simulink model "BatteryModel"  (R2025a)
settings: Solver=ode4  StartTime=startTime  StopTime=stopTime  FixedStep=600  RelTol=1e-3  EnableMultiTasking=on
PreLoadFcn:
  | load('parameters.mat'); load('temperature.mat'); load('powerDemand.mat'); ES.SoE_init = 0.5; startTime = 0; stopTime = 86400; ES.seriesCells = 84; ES.parallCells = 5;
StopFcn:
  | figure('Name', 'Battery Performance Dashboard', 'NumberTitle', 'off'); load('powerDemand.mat', 'powerDemand'); subplot(1,3,1); stairs([0:10:1430]/60, powerDemand/1e3, 'k-', 'linewidth', 2, 'DisplayName', 'Demand Track'); hold on; try stairs(tout/3600, actualPowerDrawn/1e3, 'r-', 'LineWidth', 1); catch; end; xlabel('Time [h]'); ylabel('Power [kW]'); grid on; title('Power Flux'); subplot(1,3,2); try stairs(tout/3600, esSOC*100, 'color', [0.9290 0.6940 0.1250], 'linewidth', 2); catch; end; xlabel('Time [h]'); ylim([0 110]); ylabel('% SOC'); grid on; title('Pack Energy Level'); subplot(1,3,3); try stairs(tout/3600, cellCapacity./cellCapacity(1)*100, 'k-', 'linewidth', 2); catch; end; xlabel('Time [h]'); ylabel('% SOH'); grid on; title('State of Health');
values from neighbouring files (symbols this model uses):
  ECM =     [matlab.mat]    (also in parameters.mat)
  ES =     [matlab.mat]    (also in parameters.mat)
  powerDemand = [230 3117.09108838 230 3802.27406847 230 230 230 3183.29523095 230 230 3203.47775068 230 ... (144 elements, 144x1)]    [powerDemand.mat]
  tempCelcius = [22 21.579121106 21.1646131714 20.7563616064 22.9631354938 24.9321480764 24.4525353275 23.9803499415 23.5154583277 23.0577292983 22.6070340251 22.163245997 ... (144 elements, 144x1)]    [temperature.mat]
undefined symbols (not defined in the file or in its folder): DiscIntNeverNeededParam
libraries: simulink x2
settings Model: Creator=Mario  LastModifiedBy=franc
settings SolverCC: AlgebraicLoopSolver=TrustRegion
settings DataIOCC: LimitDataPoints=on  SaveFormat=Array  SignalLoggingSaveFormat=ModelDataLogs  ReturnWorkspaceOutputs=off
settings OptimizationCC: LifeSpan=inf
settings DebuggingCC: SignalInfNanChecking=error  ReadBeforeWriteMsg=DisableAll  WriteAfterWriteMsg=DisableAll  WriteAfterReadMsg=DisableAll  InheritedTsInSrcMsg=none  MultiTaskDSMMsg=none  MultiTaskCondExecSysMsg=none  ParameterPrecisionLossMsg=none  UnconnectedInputMsg=warning  UnconnectedOutputMsg=warning  UnconnectedLineMsg=warning  AllowSymbolicDim=off  SFUnexpectedBacktrackingDiag=warning  SFNoUnconditionalDefaultTransitionDiag=warning  SFExecutionAtInitializationDiag=none  ArithmeticOperatorsInVariantConditions=warning
settings HardwareCC: ProdBitPerPointer=32.0  ProdBitPerSizeT=32.0  ProdBitPerPtrDiffT=32.0  ProdLargestAtomicFloat=None  ProdIntDivRoundTo=Undefined  ProdEndianess=Unspecified  ProdWordSize=32.0  ProdHWDeviceType=32-bit Generic
settings ModelReferenceCC: UpdateModelReferenceTargets=IfOutOfDate  EnableRefExpFcnMdlSchedulingChecks=on  PropagateSignalLabelsOutOfModel=off
settings SFSimCC: SFSimEcho=off  SimUseLocalCustomCode=off  CustomCodeUndefinedFunction=UseInterfaceOnly
settings RTWCC: RTWUseLocalCustomCode=off  GPUComputeCapability=3.5  DLArmComputeVersion=19.05
settings CodeAppCC: StateflowObjectComments=on
settings GRTTargetCC: TargetLangStandard=C89/C90 (ANSI)
settings ConfigComp: CovMetricSettings=dw  CovSaveCumulativeToWorkspaceVar=on  CovSaveSingleToWorkspaceVar=on  CovExternalEMLEnable=off  CovSFcnEnable=off

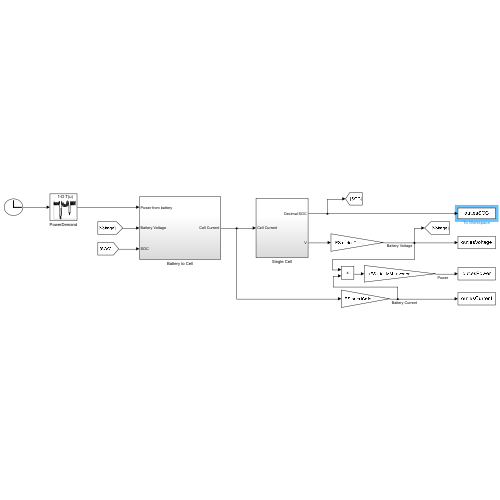
[thumbnail: Simulink's stored preview of the top-level diagram]
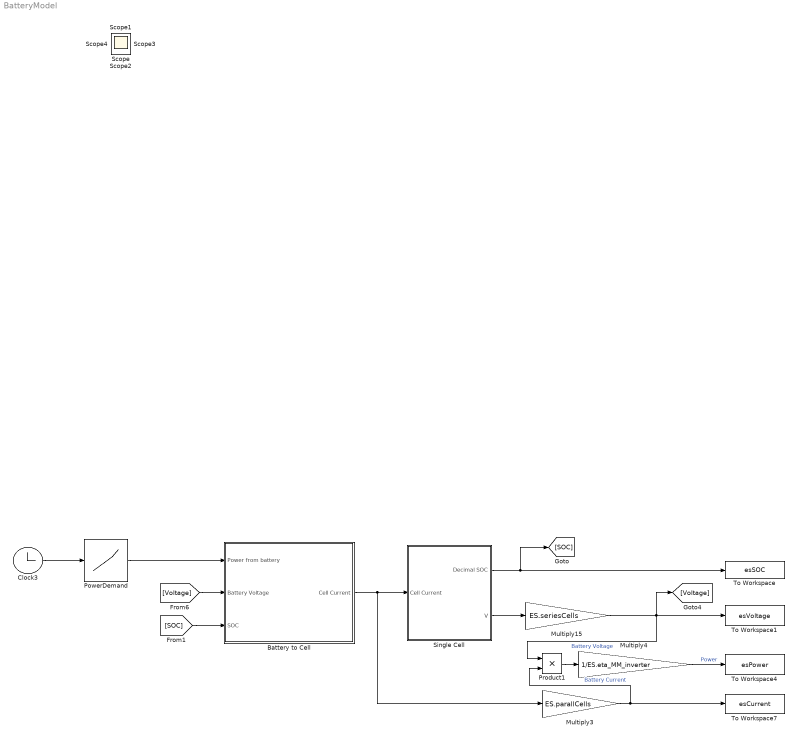
== system BatteryModel ==
  Battery to Cell : Subsystem
  Clock3 : Clock
  Multiply15 : Gain  Gain=ES.seriesCells
  Multiply3 : Gain  Gain=ES.parallCells
  Multiply4 : Gain  Gain=1/ES.eta_MM_inverter
  PowerDemand : Lookup_n-D  NumberOfTableDimensions=1  BreakpointsForDimension1=[0:600:85800]  Table=powerDemand  InternalRulePriority=Speed  RndMeth=Simplest
  Product1 : Product
  "Single Cell " : Subsystem
  To Workspace : ToWorkspace  VariableName=esSOC  SampleTime=-1
  To Workspace1 : ToWorkspace  VariableName=esVoltage  SampleTime=-1
  To Workspace4 : ToWorkspace  VariableName=esPower  SampleTime=-1
  To Workspace7 : ToWorkspace  VariableName=esCurrent  SampleTime=-1
  Scope{,1..4} (5 alike) : Scope
      Scope settings: ActiveDisplayYMinimum=-1  ActiveDisplayYMaximum=1
      Scope1 settings: ActiveDisplayYMinimum=-0.125  ActiveDisplayYMaximum=1.125  DataLoggingVariableName=ScopeData2
      Scope2 settings: ActiveDisplayYMinimum=-0.02087  ActiveDisplayYMaximum=0.18787  DataLoggingVariableName=ScopeData3
      Scope3 settings: ActiveDisplayYMinimum=-0.04167  ActiveDisplayYMaximum=0.375  DataLoggingVariableName=ScopeData4
      Scope4 settings: ActiveDisplayYMinimum=-0.04167  ActiveDisplayYMaximum=0.375  DataLoggingVariableName=ScopeData5
  wires:
  Clock3/1 -> PowerDemand/1
  Multiply4/1 -> To Workspace4/1  "Power"
  Product1/1 -> Multiply4/1
  Multiply3/1 -> Product1/2, To Workspace7/1  "Battery Current"
  Battery to Cell/1(Cell Current) -> "Single Cell "/1(Cell Current), Multiply3/1
  Multiply15/1 -> [Voltage], Product1/1, To Workspace1/1  "Battery Voltage"
  "Single Cell "/2(V) -> Multiply15/1
  "Single Cell "/1(Decimal SOC) -> [SOC], To Workspace/1
  [SOC] -> Battery to Cell/3(SOC)
  [Voltage] -> Battery to Cell/2(Battery Voltage)
  PowerDemand/1 -> Battery to Cell/1(Power from battery)

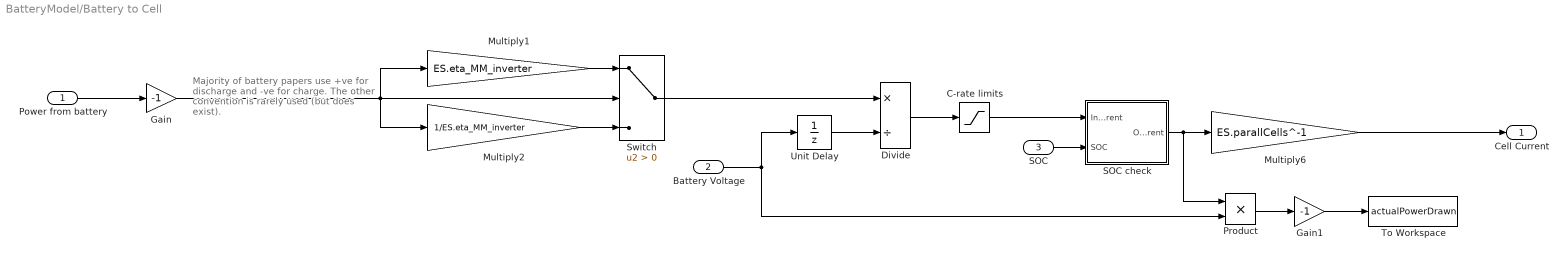
== system BatteryModel/Battery to Cell ==
  note: Majority of battery papers use
      | +ve for discharge and -ve for charge.
      |
      | The other convention is rarely used (but does exist).
  Power from battery : Inport
  Battery Voltage : Inport  Port=2
  SOC : Inport  Port=3
  C-rate limits : Saturate  UpperLimit=ES.C_Rate_maxCh*ES.battEnergy_Ah  LowerLimit=-1*ES.C_Rate_maxDisch*ES.battEnergy_Ah
  Divide : Product  Inputs=*/
  Gain : Gain  Gain=-1
  Gain1 : Gain  Gain=-1
  Multiply1 : Gain  Gain=ES.eta_MM_inverter
  Multiply2 : Gain  Gain=1/ES.eta_MM_inverter
  Multiply6 : Gain  Gain=ES.parallCells^-1
  Product : Product
  SOC check : Subsystem
  Switch : Switch  Criteria=u2 > Threshold  SaturateOnIntegerOverflow=off  InputSameDT=off
  To Workspace : ToWorkspace  VariableName=actualPowerDrawn  SampleTime=-1
  Unit Delay : UnitDelay  InitialCondition=ES.init_battVnom  SampleTime=-1  HasFrameUpgradeWarning=on
  Cell Current : Outport
  wires:
  C-rate limits/1 -> SOC check/1(InputCurrent)
  Divide/1 -> C-rate limits/1
  SOC check/1(OutputCurrent) -> Product/1, Multiply6/1
  SOC/1 -> SOC check/2(SOC)
  Unit Delay/1 -> Divide/2
  Battery Voltage/1 -> Product/2, Unit Delay/1
  Power from battery/1 -> Gain/1
  Multiply2/1 -> Switch/3
  Multiply1/1 -> Switch/1
  Product/1 -> Gain1/1
  Multiply6/1 -> Cell Current/1
  Switch/1 -> Divide/1
  Gain1/1 -> To Workspace/1
  Gain/1 -> Multiply1/1, Switch/2, Multiply2/1

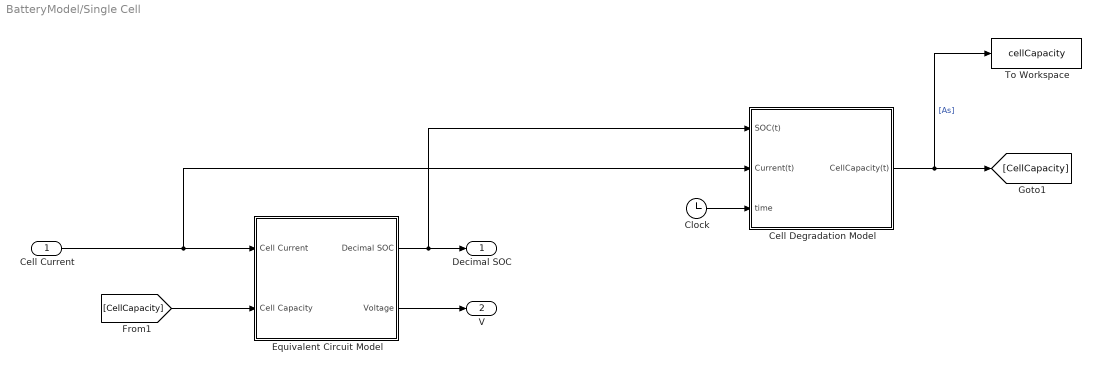
== system BatteryModel/Single Cell  ==
  Cell Current : Inport
  Cell Degradation Model : Subsystem
  Clock : Clock
  Equivalent Circuit Model : Subsystem
  To Workspace : ToWorkspace  VariableName=cellCapacity  SampleTime=-1
  Decimal SOC : Outport
  V : Outport  Port=2
  wires:
  Equivalent Circuit Model/1(Decimal SOC) -> Cell Degradation Model/1(SOC(t)), Decimal SOC/1
  Cell Degradation Model/1(CellCapacity(t)) -> To Workspace/1, [CellCapacity]  "[As]"
  [CellCapacity] -> Equivalent Circuit Model/2(Cell Capacity)
  Equivalent Circuit Model/2(Voltage) -> V/1
  Clock/1 -> Cell Degradation Model/3(time)
  Cell Current/1 -> Equivalent Circuit Model/1(Cell Current), Cell Degradation Model/2(Current(t))

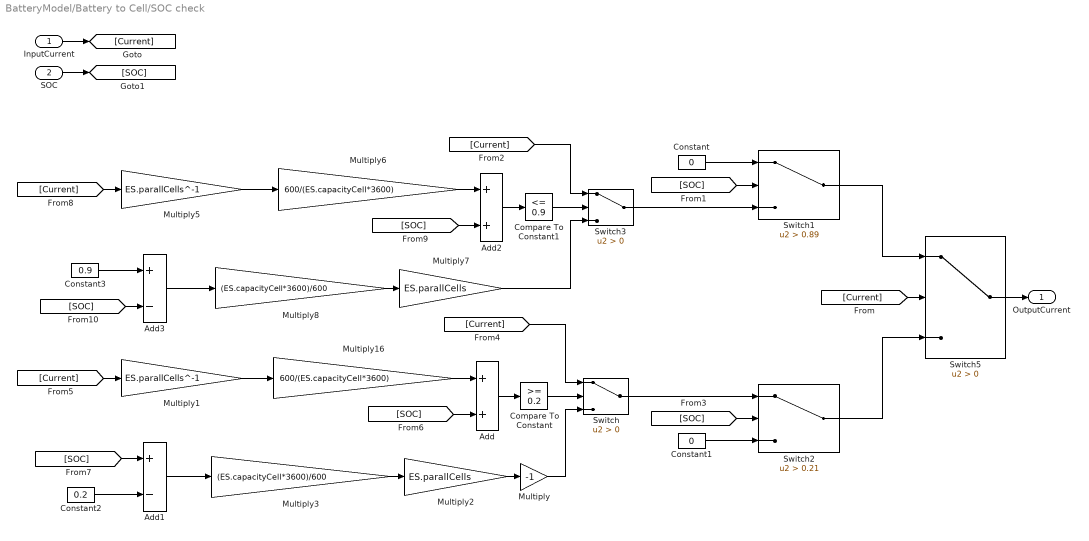
== system BatteryModel/Battery to Cell/SOC check ==
  InputCurrent : Inport
  SOC : Inport  Port=2
  Add : Sum
  Add1 : Sum  Inputs=+-
  Add2 : Sum
  Add3 : Sum  Inputs=+-
  Compare To Constant : simulink/Logic and Bit Operations/Compare To Constant  relop=>=  const=0.2  OutDataTypeStr=boolean
  Compare To Constant1 : simulink/Logic and Bit Operations/Compare To Constant  relop=<=  const=0.9  OutDataTypeStr=boolean
  Constant : Constant  Value=0
  Constant1 : Constant  Value=0
  Constant2 : Constant  Value=0.2
  Constant3 : Constant  Value=0.9
  Multiply : Gain  Gain=-1
  Multiply1 : Gain  Gain=ES.parallCells^-1
  Multiply16 : Gain  Gain=600/(ES.capacityCell*3600)
  Multiply2 : Gain  Gain=ES.parallCells
  Multiply3 : Gain  Gain=(ES.capacityCell*3600)/600
  Multiply5 : Gain  Gain=ES.parallCells^-1
  Multiply6 : Gain  Gain=600/(ES.capacityCell*3600)
  Multiply7 : Gain  Gain=ES.parallCells
  Multiply8 : Gain  Gain=(ES.capacityCell*3600)/600
  Switch : Switch  Criteria=u2 > Threshold  SaturateOnIntegerOverflow=off  InputSameDT=off
  Switch1 : Switch  Criteria=u2 > Threshold  Threshold=0.89  SaturateOnIntegerOverflow=off  InputSameDT=off
  Switch2 : Switch  Criteria=u2 > Threshold  Threshold=0.21  SaturateOnIntegerOverflow=off  InputSameDT=off
  Switch3 : Switch  Criteria=u2 > Threshold  SaturateOnIntegerOverflow=off  InputSameDT=off
  Switch5 : Switch  Criteria=u2 > Threshold  SaturateOnIntegerOverflow=off  InputSameDT=off
  OutputCurrent : Outport
  wires:
  Switch5/1 -> OutputCurrent/1
  InputCurrent/1 -> [Current]
  SOC/1 -> [SOC]
  [Current] -> Switch5/2
  [SOC] -> Switch1/2
  Constant/1 -> Switch1/1
  Switch3/1 -> Switch1/3
  Switch/1 -> Switch2/1
  Constant1/1 -> Switch2/3
  [SOC] -> Switch2/2
  Multiply/1 -> Switch/3
  Multiply2/1 -> Multiply/1
  Multiply1/1 -> Multiply16/1
  [SOC] -> Add1/1
  Multiply3/1 -> Multiply2/1
  [Current] -> Multiply1/1
  Add1/1 -> Multiply3/1
  Add/1 -> Compare To Constant/1
  Multiply16/1 -> Add/1
  Compare To Constant/1 -> Switch/2
  [SOC] -> Add/2
  Constant2/1 -> Add1/2
  Multiply7/1 -> Switch3/3
  Multiply5/1 -> Multiply6/1
  Constant3/1 -> Add3/1
  Multiply8/1 -> Multiply7/1
  [Current] -> Multiply5/1
  Add3/1 -> Multiply8/1
  Add2/1 -> Compare To Constant1/1
  Multiply6/1 -> Add2/1
  Compare To Constant1/1 -> Switch3/2
  [SOC] -> Add2/2
  [SOC] -> Add3/2
  [Current] -> Switch3/1
  Switch1/1 -> Switch5/1
  [Current] -> Switch/1
  Switch2/1 -> Switch5/3

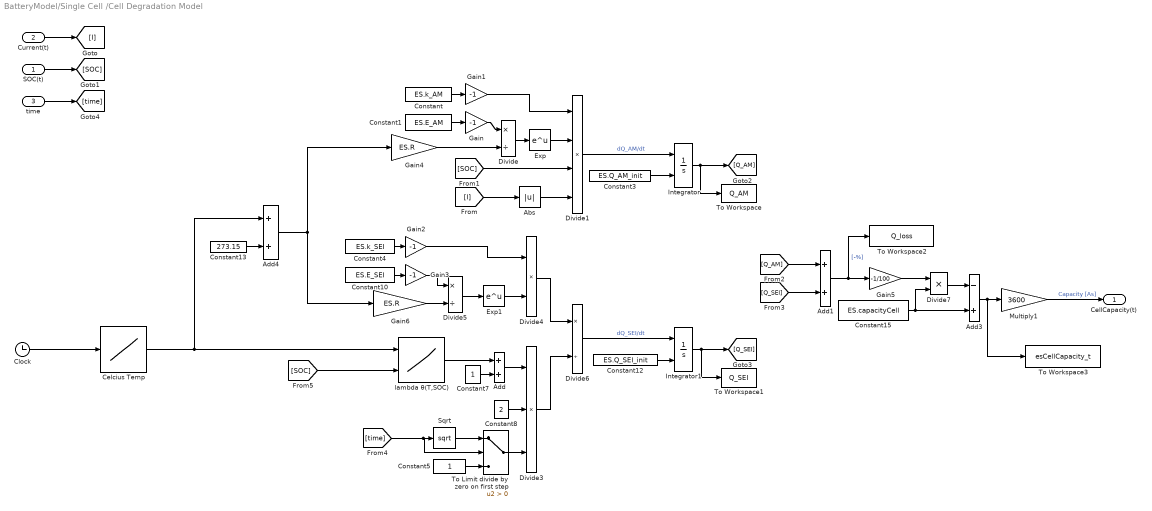
== system BatteryModel/Single Cell /Cell Degradation Model ==
  SOC(t) : Inport
  Current(t) : Inport  Port=2
  time : Inport  Port=3
  Abs : Abs  SaturateOnIntegerOverflow=off
  Add : Sum
  Add1 : Sum
  Add3 : Sum  Inputs=-+
  Add4 : Sum
  Celcius Temp : Lookup_n-D  NumberOfTableDimensions=1  BreakpointsForDimension1=[0:600:85800]  Table=tempCelcius  InternalRulePriority=Speed  RndMeth=Simplest
  Clock : Clock
  Constant : Constant  Value=ES.k_AM
  Constant1 : Constant  Value=ES.E_AM
  Constant10 : Constant  Value=ES.E_SEI
  Constant12 : Constant  Value=ES.Q_SEI_init
  Constant13 : Constant  Value=273.15
  Constant15 : Constant  Value=ES.capacityCell
  Constant3 : Constant  Value=ES.Q_AM_init
  Constant4 : Constant  Value=ES.k_SEI
  Constant5 : Constant
  Constant7 : Constant
  Constant8 : Constant  Value=2
  Divide : Product  Inputs=*/
  Divide1 : Product  Inputs=****
  Divide3 : Product  Inputs=***
  Divide4 : Product  Inputs=**
  Divide5 : Product  Inputs=*/
  Divide6 : Product  Inputs=*/
  Divide7 : Product  Inputs=**
  Exp : Math
  Exp1 : Math
  Gain{,1..3} (4 alike) : Gain  Gain=-1
  Gain4 : Gain  Gain=ES.R
  Gain5 : Gain  Gain=-1/100
  Gain6 : Gain  Gain=ES.R
  Integrator : Integrator  InitialConditionSource=external
  Integrator1 : Integrator  InitialConditionSource=external
  Multiply1 : Gain  Gain=3600
  Sqrt : Sqrt
  To Limit divide by zero on first step : Switch  Criteria=u2 > Threshold  SaturateOnIntegerOverflow=off  InputSameDT=off
  To Workspace : ToWorkspace  VariableName=Q_AM  SampleTime=-1
  To Workspace1 : ToWorkspace  VariableName=Q_SEI  SampleTime=-1
  To Workspace2 : ToWorkspace  VariableName=Q_loss  SampleTime=-1
  To Workspace3 : ToWorkspace  VariableName=esCellCapacity_t  SampleTime=-1
  lambda θ(T,SOC) : Lookup_n-D  BreakpointsForDimension1=ES.lookupT  BreakpointsForDimension2=ES.lookupSOC  Table=ES.lookupThetaLambda  InternalRulePriority=Speed  RndMeth=Simplest
      settings: InputPortMap=u0,u1
  CellCapacity(t) : Outport
  wires:
  Constant1/1 -> Gain/1
  Divide/1 -> Exp/1
  Current(t)/1 -> [I]
  SOC(t)/1 -> [SOC]
  Exp/1 -> Divide1/2
  Divide1/1 -> Integrator/1  "dQ_AM/dt"
  Constant3/1 -> Integrator/2
  Constant7/1 -> Add/2
  Constant8/1 -> Divide3/2
  [time] -> To Limit divide by zero on first step/2, Sqrt/1
  Divide3/1 -> Divide6/2
  Constant4/1 -> Gain2/1
  Add4/1 -> Gain4/1, Gain6/1
  Constant10/1 -> Gain3/1
  Divide5/1 -> Exp1/1
  Constant12/1 -> Integrator1/2
  Divide6/1 -> Integrator1/1  "dQ_SEI/dt"
  Integrator1/1 -> [Q_SEI], To Workspace1/1
  [Q_AM] -> Add1/1
  [Q_SEI] -> Add1/2
  Add1/1 -> To Workspace2/1, Gain5/1  "[-%]"
  Exp1/1 -> Divide4/2
  Divide4/1 -> Divide6/1
  [I] -> Abs/1
  Abs/1 -> Divide1/4
  time/1 -> [time]
  Sqrt/1 -> To Limit divide by zero on first step/1
  Constant5/1 -> To Limit divide by zero on first step/3
  To Limit divide by zero on first step/1 -> Divide3/3
  Celcius Temp/1 -> Add4/1, lambda θ(T,SOC)/1
  [SOC] -> lambda θ(T,SOC)/2
  Integrator/1 -> To Workspace/1, [Q_AM]
  Gain/1 -> Divide/1
  Constant/1 -> Gain1/1
  Gain1/1 -> Divide1/1
  Gain2/1 -> Divide4/1
  Gain3/1 -> Divide5/1
  lambda θ(T,SOC)/1 -> Add/1
  Add/1 -> Divide3/1
  [SOC] -> Divide1/3
  Gain5/1 -> Divide7/1
  Constant15/1 -> Divide7/2, Add3/2
  Divide7/1 -> Add3/1
  Add3/1 -> To Workspace3/1, Multiply1/1
  Multiply1/1 -> CellCapacity(t)/1  "Capacity [As]"
  Gain4/1 -> Divide/2
  Constant13/1 -> Add4/2
  Gain6/1 -> Divide5/2
  Clock/1 -> Celcius Temp/1

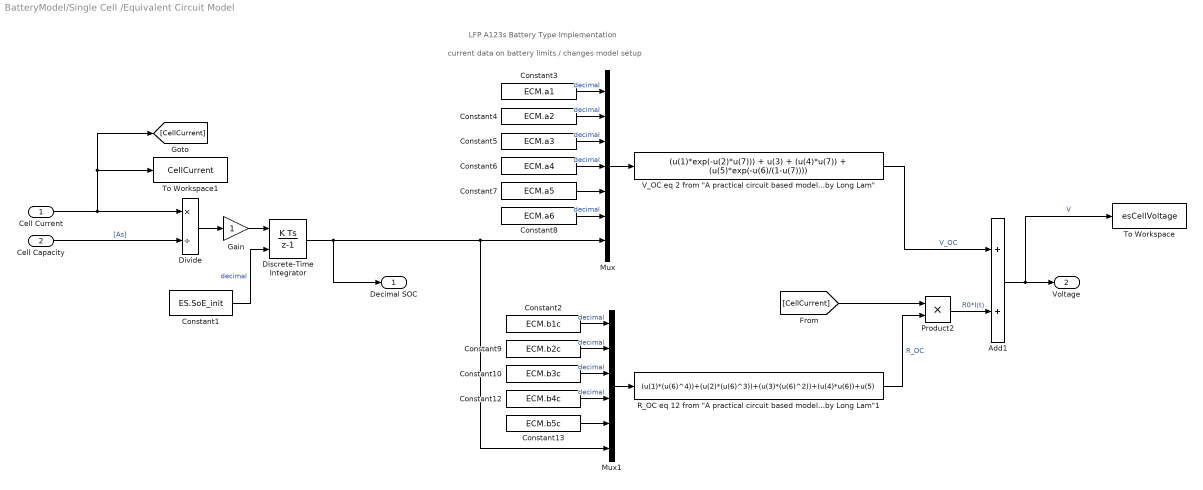
== system BatteryModel/Single Cell /Equivalent Circuit Model ==
  note: current data on battery limits / changes model setup
  note: LFP A123s Battery Type Implementation
  Cell Current : Inport
  Cell Capacity : Inport  Port=2
  Add1 : Sum
  Constant1 : Constant  Value=ES.SoE_init
  Constant10 : Constant  Value=ECM.b3c
  Constant12 : Constant  Value=ECM.b4c
  Constant13 : Constant  Value=ECM.b5c
  Constant2 : Constant  Value=ECM.b1c
  Constant3 : Constant  Value=ECM.a1
  Constant4 : Constant  Value=ECM.a2
  Constant5 : Constant  Value=ECM.a3
  Constant6 : Constant  Value=ECM.a4
  Constant7 : Constant  Value=ECM.a5
  Constant8 : Constant  Value=ECM.a6
  Constant9 : Constant  Value=ECM.b2c
  Discrete-Time Integrator : DiscreteIntegrator  InitialConditionSource=external  SampleTime=-1  ICPrevOutput=DiscIntNeverNeededParam  ICPrevScaledInput=DiscIntNeverNeededParam
  Divide : Product  Inputs=*/
  Gain : Gain
  Mux : Mux  Inputs=7
  Mux1 : Mux  Inputs=6
  Product2 : Product
  "R_OC eq 12 from \"A practical circuit based model...by Long Lam\"1" : Fcn  Expr=(u(1)*(u(6)^4))+(u(2)*(u(6)^3))+(u(3)*(u(6)^2))+(u(4)*u(6))+u(5)
  To Workspace : ToWorkspace  VariableName=esCellVoltage  SampleTime=-1
  To Workspace1 : ToWorkspace  VariableName=CellCurrent  SampleTime=-1
  "V_OC eq 2 from \"A practical circuit based model...by Long Lam\"" : Fcn  Expr=(u(1)*exp(-u(2)*u(7))) + u(3) + (u(4)*u(7)) + (u(5)*exp(-u(6)/(1-u(7))))
  Decimal SOC : Outport
  Voltage : Outport  Port=2
  wires:
  Discrete-Time Integrator/1 -> Mux/7, Mux1/6, Decimal SOC/1
  Divide/1 -> Gain/1
  Cell Current/1 -> Divide/1, [CellCurrent], To Workspace1/1
  Constant1/1 -> Discrete-Time Integrator/2  "decimal"
  Cell Capacity/1 -> Divide/2  "[As]"
  Product2/1 -> Add1/2  "R0*I(t)"
  Add1/1 -> To Workspace/1, Voltage/1  "V"
  Constant7/1 -> Mux/5
  Constant3/1 -> Mux/1  "decimal"
  Constant4/1 -> Mux/2  "decimal"
  Constant5/1 -> Mux/3  "decimal"
  Constant6/1 -> Mux/4  "decimal"
  Constant8/1 -> Mux/6  "decimal"
  Mux/1 -> "V_OC eq 2 from \"A practical circuit based model...by Long Lam\""/1
  "V_OC eq 2 from \"A practical circuit based model...by Long Lam\""/1 -> Add1/1  "V_OC"
  Constant12/1 -> Mux1/4  "decimal"
  Mux1/1 -> "R_OC eq 12 from \"A practical circuit based model...by Long Lam\"1"/1
  Constant10/1 -> Mux1/3  "decimal"
  Constant9/1 -> Mux1/2  "decimal"
  Constant2/1 -> Mux1/1  "decimal"
  Constant13/1 -> Mux1/5
  "R_OC eq 12 from \"A practical circuit based model...by Long Lam\"1"/1 -> Product2/2  "R_OC"
  [CellCurrent] -> Product2/1
  Gain/1 -> Discrete-Time Integrator/1
